simulink model "HIL_Testing_SW"  (Simulink 7.5)
settings: Solver=ode1  StartTime=0.0  StopTime=Inf  FixedStep=0.001  RelTol=1e-3
PostLoadFcn:
  | , if any(exist('dsrtsu_mdlpostloadfcn', 'file') == [2, 3, 6]), try dsrtsu_mdlpostloadfcn('Execute', bdroot); catch fprintf('Error in PostLoadFcn (dsrtsu_mdlpostloadfcn) for model "%s":\n %s\n', bdroot, lasterr); end, end,
undefined symbols (not defined in the file): CeBSER_Cnt_NumTempAxisPts, ChargeCord, ChargeCord_Control, ChargeToSOCCurr, ChrgCurrLim, CrntSens1Fine, CS_SOCSetPt, CyclerMaxChrgPwr, CyclerMaxDschrgPwr, deltaAhr, Drive_1, Drive_10, Drive_11, Drive_12, Drive_13, Drive_14, Drive_15, Drive_16, Drive_17, Drive_18, Drive_19, Drive_2, Drive_20, Drive_21, Drive_22, Drive_23, Drive_24, Drive_25, Drive_26, Drive_27, Drive_28, Drive_29, Drive_3, Drive_30, Drive_31, Drive_32, Drive_33, Drive_34, Drive_35, Drive_36, Drive_37, Drive_38, Drive_39, Drive_4, Drive_40, Drive_41, Drive_42, Drive_43, Drive_44, Drive_45, Drive_46, Drive_47, Drive_48, Drive_49, Drive_5, Drive_50, Drive_51, Drive_6, Drive_7, Drive_8 ... (+50)
libraries: simulink x129, rtican x50, rti2211sailib x5, rti2211serlib x5, rti2202miolib x3
(part 18 of 23)

== system HIL_Testing_SW/LionsHeart/FeaturePresentation/Down_to_Business/DriveProfile_ModeControl/Pulse ==
  Current : Inport  OutDataType=fixdt(1, 16)  OutScaling=2^0
  Voltage : Inport  Port=2  OutDataType=fixdt(1, 16)  OutScaling=2^0
  Direction : Inport  Port=3  OutDataType=fixdt(1, 16)  OutScaling=2^0
  Enable : EnablePort  StatesWhenEnabling=reset
  Data Store Read1 : DataStoreRead  DataStoreName=CyclerMaxDschrgPwr  SampleTime=0
  Data Store Read10 : DataStoreRead  DataStoreName=DschrgCurrLim  SampleTime=0
  Data Store Read2 : DataStoreRead  DataStoreName=CyclerMaxChrgPwr  SampleTime=0
  Data Store Read9 : DataStoreRead  DataStoreName=ChrgCurrLim  SampleTime=0
  Data Type Conversion : DataTypeConversion  OutDataTypeMode=single  OutDataType=sfix(16)  OutScaling=2^0  OutDataTypeStr=single
  Data Type Conversion1 : DataTypeConversion  OutDataTypeMode=single  OutDataType=sfix(16)  OutScaling=2^0  OutDataTypeStr=single
  Pulse : Stateflow chart  TreatAsAtomicUnit=on
  PulseDuration : Constant  Tag=R12-1  Value=10  OutDataTypeMode=double  OutDataType=sfix(16)  OutScaling=2^0  OutDataTypeStr=double
  Terminator2 : Terminator
  simstep : Constant  Tag=R12-1  Value=SimStep_dT  OutDataTypeMode=double  OutDataType=sfix(16)  OutScaling=2^0  OutDataTypeStr=double
  Profile_Data_Pulse : Outport  OutDataType=sfix(16)  OutScaling=2^0
  Mode_Cntrl : Outport  Port=2  OutDataType=sfix(16)  OutScaling=2^0
  PulseStep : Outport  Port=3  OutDataType=sfix(16)  OutScaling=2^0
  wires:
  Current/1 -> [Current]
  Voltage/1 -> [Voltage]
  [Voltage] -> Pulse/1(Voltage)
  [Current] -> Pulse/2(Current)
  simstep/1 -> Data Type Conversion1/1
  Data Type Conversion/1 -> Profile_Data_Pulse/1
  Pulse/3(Mode_Cntrl) -> Mode_Cntrl/1
  Pulse/1(Control_Value) -> Data Type Conversion/1
  Data Type Conversion1/1 -> Pulse/3(sim_step_time)
  Pulse/2(WaitTime) -> Terminator2/1  "Waitime"
  Data Store Read9/1 -> Pulse/4(ChrgCurrLim)
  Data Store Read10/1 -> Pulse/5(DischrgCurrLim)
  Pulse/4(Step) -> PulseStep/1
  Direction/1 -> [direction]
  [direction] -> Pulse/6(Direction)
  Data Store Read1/1 -> Pulse/8(DPower)
  Data Store Read2/1 -> Pulse/7(CPower)
  PulseDuration/1 -> Pulse/9(PulseDuration)

== system HIL_Testing_SW/LionsHeart/FeaturePresentation/Down_to_Business/DriveProfile_ModeControl/Rate ==
  CurrLimit : Inport  OutDataType=fixdt(1, 16)  OutScaling=2^0
  Rate : Inport  Port=2  OutDataType=fixdt(1, 16)  OutScaling=2^0
  Direction : Inport  Port=3  OutDataType=fixdt(1, 16)  OutScaling=2^0
  Enable : EnablePort  StatesWhenEnabling=reset
  Data Store Read10 : DataStoreRead  DataStoreName=DisChrgCurr_Limit  SampleTime=0
  Data Store Read9 : DataStoreRead  DataStoreName=ChargeLimit_Temp  SampleTime=0
  Data Store Write15 : DataStoreWrite  DataStoreName=ChrgCurrLim  SampleTime=-1
  Data Store Write16 : DataStoreWrite  DataStoreName=DschrgCurrLim  SampleTime=-1
  Data Type Conversion1 : DataTypeConversion  OutDataTypeMode=single  OutDataType=sfix(16)  OutScaling=2^0  OutDataTypeStr=single
  PTime : Constant  Value=4  OutDataTypeMode=single  OutDataType=fixdt(1, 16)  OutScaling=2^0  OutDataTypeStr=single
  Product : Product  OutDataType=fixdt(1, 16)  OutScaling=2^0  RndMeth=Zero
  PulseRate : Stateflow chart  TreatAsAtomicUnit=on
  Rate Limiter Dynamic1 : simulink/Discontinuities/Rate Limiter Dynamic  SystemSampleTime=-1
  Rate Limiter Dynamic2 : simulink/Discontinuities/Rate Limiter Dynamic  SystemSampleTime=-1
  Saturation Dynamic : simulink/Discontinuities/Saturation Dynamic  SystemSampleTime=-1  OutMin=[]  OutMax=[]  OutDataTypeStr=single  OutputDataTypeScalingMode=single  OutDataType=sfix(16)  OutScaling=2^-10  DoSatur=off
  Saturation Dynamic1 : simulink/Discontinuities/Saturation Dynamic  SystemSampleTime=-1  OutMin=[]  OutMax=[]  OutDataTypeStr=single  OutputDataTypeScalingMode=single  OutDataType=sfix(16)  OutScaling=2^-10  DoSatur=off
  lolim : Constant  Value=0  OutDataTypeMode=single  OutDataType=fixdt(1, 16)  OutScaling=2^0  OutDataTypeStr=single
  lolim1 : Constant  Value=0  OutDataTypeMode=single  OutDataType=fixdt(1, 16)  OutScaling=2^0  OutDataTypeStr=single
  lolim2 : Constant  Value=-1  OutDataTypeMode=single  OutDataType=fixdt(1, 16)  OutScaling=2^0  OutDataTypeStr=single
  simstep : Constant  Tag=R12-1  Value=SimStep_dT  OutDataTypeMode=double  OutDataType=sfix(16)  OutScaling=2^0  OutDataTypeStr=double
  Profile_Data_rate : Outport  OutDataType=sfix(16)  OutScaling=2^0
  Mode_Cntrl_rate : Outport  Port=2  OutDataType=sfix(16)  OutScaling=2^0
  RateStep : Outport  Port=3  OutDataType=sfix(16)  OutScaling=2^0
  wires:
  Data Type Conversion1/1 -> PulseRate/1(sim_step_time)
  simstep/1 -> Data Type Conversion1/1
  Rate Limiter Dynamic1/1 -> Saturation Dynamic/2
  CurrLimit/1 -> [CurrLimit]
  Rate/1 -> [Rate]
  PulseRate/1(Control_Value) -> Profile_Data_rate/1
  PulseRate/3(Mode_Cntrl) -> Mode_Cntrl_rate/1
  PulseRate/4(Step) -> RateStep/1
  Data Store Read9/1 -> PulseRate/2(ChrgCurrLim_Cal)
  Data Store Read10/1 -> PulseRate/3(DischrgCurrLim_Cal)
  Saturation Dynamic/1 -> Data Store Write15/1
  PulseRate/2(ChrgCurrLim_Temp) -> Saturation Dynamic/1, Rate Limiter Dynamic1/2
  lolim/1 -> Rate Limiter Dynamic1/3, Saturation Dynamic/3
  [Rate] -> Rate Limiter Dynamic1/1
  Direction/1 -> PulseRate/4(Direction)
  PTime/1 -> PulseRate/5(PTime)
  [CurrLimit] -> PulseRate/6(CurrLim)
  Rate Limiter Dynamic2/1 -> Saturation Dynamic1/2
  PulseRate/5(DischrgCurrLim_Temp) -> Rate Limiter Dynamic2/2, Saturation Dynamic1/1
  lolim1/1 -> Rate Limiter Dynamic2/3, Saturation Dynamic1/3
  lolim2/1 -> Product/1
  Saturation Dynamic1/1 -> Product/2
  Product/1 -> Data Store Write16/1
  [Rate] -> Rate Limiter Dynamic2/1

== system HIL_Testing_SW/LionsHeart/FeaturePresentation/Down_to_Business/DriveProfile_ModeControl/Standby_Sub ==
  Enable : EnablePort
  Standby : Constant  Value=single(3)  OutDataType=sfix(16)  OutScaling=2^0
  Standby1 : Outport  OutDataType=fixdt(1, 16)  OutScaling=2^0
  wires:
  Standby/1 -> Standby1/1

== system HIL_Testing_SW/LionsHeart/Input Processing/Voltage Processing/ChargeTermVoltage/ConvCellToPack_Volt1 ==
  note: ConvCellToPack_Volt
  CellLevel_Volt : Inport  OutDataType=sfix(16)  OutScaling=2^0
  Product : Product  OutDataType=sfix(16)  OutScaling=2^0  RndMeth=Zero
  SOCTerm : DataStoreRead  DataStoreName=NumberOfCells  SampleTime=0
  PackLevel_Volt : Outport  OutDataType=sfix(16)  OutScaling=2^0
  wires:
  SOCTerm/1 -> Product/2
  Product/1 -> PackLevel_Volt/1
  CellLevel_Volt/1 -> Product/1

== system HIL_Testing_SW/LionsHeart/Input Processing/Voltage Processing/ChargeTermVoltage/ConvCellToPack_Volt2 ==
  note: ConvCellToPack_Volt
  CellLevel_Volt : Inport  OutDataType=sfix(16)  OutScaling=2^0
  Product : Product  OutDataType=sfix(16)  OutScaling=2^0  RndMeth=Zero
  SOCTerm : DataStoreRead  DataStoreName=NumberOfCells  SampleTime=0
  PackLevel_Volt : Outport  OutDataType=sfix(16)  OutScaling=2^0
  wires:
  CellLevel_Volt/1 -> Product/1
  Product/1 -> PackLevel_Volt/1
  SOCTerm/1 -> Product/2

== system HIL_Testing_SW/LionsHeart/Input Processing/Voltage Processing/ChargeTermVoltage/LookupChrgVoltageSetPoint_BSE ==
  note: LookupChrgVoltageSetPoint
  SocACChrg : Inport  OutDataType=sfix(16)  OutScaling=2^0
  T : Inport  Port=2  OutDataType=sfix(16)  OutScaling=2^0
  Constant Value : Constant  Value=CeBSER_Cnt_NumTempAxisPts  OutDataType=sfix(16)  OutScaling=2^0
  Constant Value1 : Constant  Value=single(100)  OutDataType=sfix(16)  OutScaling=2^0
  KnBSEM_T_TempAxis : Constant  Value=KnBSEM_T_TempAxis  OutDataType=sfix(16)  OutScaling=2^0
      settings: CopyFcn=try,set_param(gcb,'Value',get_param(gcb,'Name'));catch,err=lasterror;if (isempty(strfind(err.message,'Attempting to override parameters')) || isempty(strfind(err.message,'which is inside a library link'))) rethrow(err);end;end  NameChangeFcn=try,set_param(gcb,'Value',get_param(gcb,'Name'));catch,[msgstr msgid]=lasterr;errordlg(['error ',num2str(msgid),' - ',msgstr],'Error','modal');end  OpenFcn=global edarrcal; edarrcal.cb = gcb; edfigarrcal('fig');
  Merge : Merge  Inputs=8
  Product1 : Product  Inputs=*/  OutDataType=sfix(16)  OutScaling=2^0  RndMeth=Zero
  Stateflow Chart1 : Stateflow chart  TreatAsAtomicUnit=on
      settings: CopyFcn=breaklink(gcb)
  Switch Case : SwitchCase  CaseConditions={1,2,3,4,5,6,7,8}  ShowDefaultCase=off
      settings: CopyFcn=breaklink(gcb)
  Switch Case Action Subsystem : Subsystem  TreatAsAtomicUnit=on
      settings: CopyFcn=breaklink(gcb)  PropExecContextOutsideSubsystem=on
  Switch Case Action Subsystem1 : Subsystem  TreatAsAtomicUnit=on
      settings: CopyFcn=breaklink(gcb)  PropExecContextOutsideSubsystem=on
  Switch Case Action Subsystem2 : Subsystem  TreatAsAtomicUnit=on
      settings: CopyFcn=breaklink(gcb)  PropExecContextOutsideSubsystem=on
  Switch Case Action Subsystem3 : Subsystem  TreatAsAtomicUnit=on
      settings: CopyFcn=breaklink(gcb)  PropExecContextOutsideSubsystem=on
  Switch Case Action Subsystem4 : Subsystem  TreatAsAtomicUnit=on
      settings: CopyFcn=breaklink(gcb)  PropExecContextOutsideSubsystem=on
  Switch Case Action Subsystem5 : Subsystem  TreatAsAtomicUnit=on
      settings: CopyFcn=breaklink(gcb)  PropExecContextOutsideSubsystem=on
  Switch Case Action Subsystem6 : Subsystem  TreatAsAtomicUnit=on
      settings: CopyFcn=breaklink(gcb)  PropExecContextOutsideSubsystem=on
  Switch Case Action Subsystem7 : Subsystem  TreatAsAtomicUnit=on
      settings: CopyFcn=breaklink(gcb)  PropExecContextOutsideSubsystem=on
  Output Parameter : Outport  OutDataType=sfix(16)  OutScaling=2^0
  wires:
  SocACChrg/1 -> Product1/1
  Product1/1 -> [SOC]
  Constant Value1/1 -> Product1/2
  Switch Case Action Subsystem7/1(Output Parameter) -> Merge/8
  Switch Case Action Subsystem6/1(Output Parameter) -> Merge/7
  Switch Case Action Subsystem5/1(Output Parameter) -> Merge/6
  Switch Case Action Subsystem4/1(Output Parameter) -> Merge/5
  Switch Case Action Subsystem3/1(Output Parameter) -> Merge/4
  Switch Case Action Subsystem2/1(Output Parameter) -> Merge/3
  Switch Case Action Subsystem1/1(Output Parameter) -> Merge/2
  Switch Case Action Subsystem/1(Output Parameter) -> Merge/1
  T/1 -> Stateflow Chart1/1(VeBSER_T_HV_BatTemp)
  [Idx8] -> Switch Case Action Subsystem7/Action
  [SOC] -> Switch Case Action Subsystem7/1(SOC)
  [SF] -> Switch Case Action Subsystem7/2(SF)
  [Idx7] -> Switch Case Action Subsystem6/Action
  [SOC] -> Switch Case Action Subsystem6/1(SOC)
  [SF] -> Switch Case Action Subsystem6/2(SF)
  [Idx6] -> Switch Case Action Subsystem5/Action
  [SOC] -> Switch Case Action Subsystem5/1(SOC)
  [SF] -> Switch Case Action Subsystem5/2(SF)
  [Idx5] -> Switch Case Action Subsystem4/Action
  [SOC] -> Switch Case Action Subsystem4/1(SOC)
  [SF] -> Switch Case Action Subsystem4/2(SF)
  [Idx4] -> Switch Case Action Subsystem3/Action
  [SOC] -> Switch Case Action Subsystem3/1(SOC)
  [SF] -> Switch Case Action Subsystem3/2(SF)
  [Idx3] -> Switch Case Action Subsystem2/Action
  [SOC] -> Switch Case Action Subsystem2/1(SOC)
  [SF] -> Switch Case Action Subsystem2/2(SF)
  [Idx2] -> Switch Case Action Subsystem1/Action
  [SOC] -> Switch Case Action Subsystem1/1(SOC)
  [SF] -> Switch Case Action Subsystem1/2(SF)
  Merge/1 -> Output Parameter/1
  [Idx1] -> Switch Case Action Subsystem/Action
  Switch Case/8 -> [Idx8]
  Switch Case/7 -> [Idx7]
  Switch Case/6 -> [Idx6]
  Switch Case/5 -> [Idx5]
  Switch Case/4 -> [Idx4]
  Switch Case/3 -> [Idx3]
  Switch Case/2 -> [Idx2]
  Switch Case/1 -> [Idx1]
  Stateflow Chart1/1(LeBSER_i_Indx) -> Switch Case/1
  KnBSEM_T_TempAxis/1 -> Stateflow Chart1/2(KnBSEM_T_TempAxis)
  Stateflow Chart1/2(LeBSER_r_ScaleFctr) -> [SF]
  [SOC] -> Switch Case Action Subsystem/1(SOC)
  [SF] -> Switch Case Action Subsystem/2(SF)
  Constant Value/1 -> Stateflow Chart1/3(CeBSER_Cnt_NumTempAxisPts)

== system HIL_Testing_SW/LionsHeart/Input Processing/Voltage Processing/PackVLid/ConvCellToPack_Volt4 ==
  note: ConvCellToPack_Volt
  CellLevel_Volt : Inport  OutDataType=sfix(16)  OutScaling=2^0
  NumberOfCells : DataStoreRead  DataStoreName=NumberOfCells  SampleTime=0
  Product : Product  OutDataType=sfix(16)  OutScaling=2^0  RndMeth=Zero
  PackLevel_Volt : Outport  OutDataType=sfix(16)  OutScaling=2^0
  wires:
  CellLevel_Volt/1 -> Product/1
  Product/1 -> PackLevel_Volt/1
  NumberOfCells/1 -> Product/2

== system HIL_Testing_SW/LionsHeart/Input Processing/Voltage Processing/PackVfloor/ConvCellToPack_Volt3 ==
  note: ConvCellToPack_Volt
  CellLevel_Volt : Inport  OutDataType=sfix(16)  OutScaling=2^0
  NumberOfCells : DataStoreRead  DataStoreName=NumberOfCells  SampleTime=0
  Product : Product  OutDataType=sfix(16)  OutScaling=2^0  RndMeth=Zero
  PackLevel_Volt : Outport  OutDataType=sfix(16)  OutScaling=2^0
  wires:
  NumberOfCells/1 -> Product/2
  Product/1 -> PackLevel_Volt/1
  CellLevel_Volt/1 -> Product/1

== system HIL_Testing_SW/LionsHeart/Input Processing/Voltage Processing/PackVfloor/EREV ==
  MinCellOffset : Inport  OutDataType=fixdt(1, 16)  OutScaling=2^0
  MinSectionOffset : Inport  Port=2  OutDataType=fixdt(1, 16)  OutScaling=2^0
  Enable : EnablePort
  Data Store Read : DataStoreRead  DataStoreName=MinSectionorMinCellOffset_EREV  SampleTime=0
  Switch1 : Switch  Threshold=.5  OutDataType=fixdt(1, 16)  OutScaling=2^0
  VoltageFloorOffset_EREV : Outport  OutDataType=fixdt(1, 16)  OutScaling=2^0
  wires:
  MinCellOffset/1 -> Switch1/1
  MinSectionOffset/1 -> Switch1/3
  Switch1/1 -> VoltageFloorOffset_EREV/1
  Data Store Read/1 -> Switch1/2

== system HIL_Testing_SW/LionsHeart/Input Processing/Voltage Processing/PackVfloor/Subsystem1 ==
  MinCellOffset : Inport  OutDataType=fixdt(1, 16)  OutScaling=2^0
  Enable : EnablePort
  VoltageFloorOffset : Outport  OutDataType=fixdt(1, 16)  OutScaling=2^0
  wires:
  MinCellOffset/1 -> VoltageFloorOffset/1

== system HIL_Testing_SW/RTI Data/RTI Data Store/RTI Data Store/RTI Data Store/RTI Data Store ==

== system HIL_Testing_SW/RX/Read EREV/Read HVEM/Current/Enabled Subsystem ==
  SensTwo : Inport  OutDataType=sfix(16)  OutScaling=2^0
  SensOne : Inport  Port=2  OutDataType=sfix(16)  OutScaling=2^0
  Enable : EnablePort
  Abs : Abs  OutDataType=fixdt(1, 16)  OutScaling=2^0
  Switch : Switch  Threshold=20  OutDataType=sfix(16)  OutScaling=2^0
  Out1 : Outport  OutDataType=sfix(16)  OutScaling=2^0
  wires:
  SensTwo/1 -> Switch/1
  Switch/1 -> Out1/1
  SensOne/1 -> Switch/3, Abs/1
  Abs/1 -> Switch/2

== system HIL_Testing_SW/RX/Read EREV/Read HVEM/Current/Enabled Subsystem1 ==
  SensTwo : Inport  OutDataType=sfix(16)  OutScaling=2^0
  SensOne : Inport  Port=2  OutDataType=sfix(16)  OutScaling=2^0
  Enable : EnablePort
  Abs : Abs  OutDataType=fixdt(1, 16)  OutScaling=2^0
  Switch : Switch  Threshold=20  OutDataType=sfix(16)  OutScaling=2^0
  Out1 : Outport  OutDataType=sfix(16)  OutScaling=2^0
  wires:
  Switch/1 -> Out1/1
  SensOne/1 -> Switch/1
  SensTwo/1 -> Switch/3, Abs/1
  Abs/1 -> Switch/2

== system HIL_Testing_SW/RX/Read EREV/Read HVEM/Sum of Cells/Subsystem ==
  In1 : Inport  OutDataType=fixdt(1, 16)  OutScaling=2^0
  Bus Creator : BusCreator  Inputs=42
  Bus Creator1 : BusCreator  Inputs=24
  Bus Creator2 : BusCreator  Inputs=30
  Bus Selector : BusSelector  OutputSignals=signal1.HVBatCell_003,signal1.HVBatCell_006,signal1.HVBatCell_009,signal1.HVBatCell_012,signal1.HVBatCell_015,signal1.HVBatCell_018,signal1.HVBatCell_021,signal1.HVBatCell_024,signal1.HVBatCell_002,signal1.HVBatCell_005,signal1.HVBatCell_008,signal1.HVBatCell_011,signal1.HVBatCell_014,signal1.HVBatCell_017,signal1.HVBatCell_020,signal1.HVBatCell_023,signal1.HVBatCell_001,signal1.HVBatCell_004,signal1.HVBatCell_007,signal1.HVBatCell_010,signal1.HVBatCell_013,signal1.HVBatCell_016,signal1.HVBatCell_019,signal1.HVBatCell_022,signal2.HVBatCell_027,signal2.HVBatCell_030,signal2.HVBatCell_033,signal2.HVBatCell_036,signal2.HVBatCell_039,signal2.HVBatCell_042,signal2.HVBatCell_026,signal2.HVBatCell_029,signal2.HVBatCell_032,signal2.HVBatCell_035,signal2.HVBatCell_038,signal2.HVBatCell_041,signal2.HVBatCell_025,signal2.HVBatCell_028,signal2.HVBatCell_031,signal2.HVBatCell_034,signal2.HVBatCell_037,signal2.HVBatCell_040
  Bus Selector1 : BusSelector  OutputSignals=signal2.HVBatCell_045,signal2.HVBatCell_048,signal2.HVBatCell_044,signal2.HVBatCell_047,signal2.HVBatCell_043,signal2.HVBatCell_046,signal3.HVBatCell_051,signal3.HVBatCell_054,signal3.HVBatCell_057,signal3.HVBatCell_060,signal3.HVBatCell_063,signal3.HVBatCell_066,signal3.HVBatCell_050,signal3.HVBatCell_053,signal3.HVBatCell_056,signal3.HVBatCell_059,signal3.HVBatCell_062,signal3.HVBatCell_065,signal3.HVBatCell_049,signal3.HVBatCell_052,signal3.HVBatCell_055,signal3.HVBatCell_058,signal3.HVBatCell_061,signal3.HVBatCell_064
  Bus Selector2 : BusSelector  OutputSignals=signal3.HVBatCell_069,signal3.HVBatCell_072,signal3.HVBatCell_068,signal3.HVBatCell_071,signal3.HVBatCell_067,signal3.HVBatCell_070,signal4.HVBatCell_075,signal4.HVBatCell_078,signal4.HVBatCell_081,signal4.HVBatCell_084,signal4.HVBatCell_087,signal4.HVBatCell_090,signal4.HVBatCell_093,signal4.HVBatCell_096,signal4.HVBatCell_074,signal4.HVBatCell_077,signal4.HVBatCell_080,signal4.HVBatCell_083,signal4.HVBatCell_086,signal4.HVBatCell_089,signal4.HVBatCell_092,signal4.HVBatCell_095,signal4.HVBatCell_073,signal4.HVBatCell_076,signal4.HVBatCell_079,signal4.HVBatCell_082,signal4.HVBatCell_085,signal4.HVBatCell_088,signal4.HVBatCell_091,signal4.HVBatCell_094
  Divide : Product  Inputs=*/  OutDataType=fixdt(1, 16)  OutScaling=2^-10
  Divide1 : Product  Inputs=*/  OutDataType=fixdt(1, 16)  OutScaling=2^-10
  Divide2 : Product  Inputs=*/  OutDataType=fixdt(1, 16)  OutScaling=2^-10
  MinMax : MinMax  Inputs=3  OutDataType=fixdt(1, 16)  OutScaling=2^0
  NumCells : Constant  Value=42  OutDataType=fixdt(1, 16)  OutScaling=2^0
  NumCells1 : Constant  Value=24  OutDataType=fixdt(1, 16)  OutScaling=2^0
  NumCells2 : Constant  Value=30  OutDataType=fixdt(1, 16)  OutScaling=2^0
  NumOfCells : DataStoreRead  DataStoreName=NumberOfCells  SampleTime=0
  Product : Product  OutDataType=fixdt(1, 16)  OutScaling=2^0  RndMeth=Zero
  Product1 : Product  OutDataType=fixdt(1, 16)  OutScaling=2^0  RndMeth=Zero
  Product2 : Product  OutDataType=fixdt(1, 16)  OutScaling=2^0  RndMeth=Zero
  Sum : Sum  Inputs=+  OutDataType=fixdt(1, 16)  OutScaling=2^-10
  Sum1 : Sum  Inputs=+  OutDataType=fixdt(1, 16)  OutScaling=2^-10
  Sum2 : Sum  Inputs=+  OutDataType=fixdt(1, 16)  OutScaling=2^-10
  MinSection_PackEquivalent : Outport  OutDataType=fixdt(1, 16)  OutScaling=2^0
  wires:
  In1/1 -> Bus Selector/1, Bus Selector1/1, Bus Selector2/1
  Bus Creator/1 -> Sum/1
  Sum/1 -> Divide/1
  NumCells/1 -> Divide/2
  Divide/1 -> Product/1
  Bus Selector/1 -> Bus Creator/1  "<HVBatCell_003>"
  Bus Selector/2 -> Bus Creator/2  "<HVBatCell_006>"
  Bus Selector/3 -> Bus Creator/3  "<HVBatCell_009>"
  Bus Selector/4 -> Bus Creator/4  "<HVBatCell_012>"
  Bus Selector/5 -> Bus Creator/5  "<HVBatCell_015>"
  Bus Selector/6 -> Bus Creator/6  "<HVBatCell_018>"
  Bus Selector/7 -> Bus Creator/7  "<HVBatCell_021>"
  Bus Selector/8 -> Bus Creator/8  "<HVBatCell_024>"
  Bus Selector/9 -> Bus Creator/9  "<HVBatCell_002>"
  Bus Selector/10 -> Bus Creator/10  "<HVBatCell_005>"
  Bus Selector/11 -> Bus Creator/11  "<HVBatCell_008>"
  Bus Selector/12 -> Bus Creator/12  "<HVBatCell_011>"
  Bus Selector/13 -> Bus Creator/13  "<HVBatCell_014>"
  Bus Selector/14 -> Bus Creator/14  "<HVBatCell_017>"
  Bus Selector/15 -> Bus Creator/15  "<HVBatCell_020>"
  Bus Selector/16 -> Bus Creator/16  "<HVBatCell_023>"
  Bus Selector/17 -> Bus Creator/17  "<HVBatCell_001>"
  Bus Selector/18 -> Bus Creator/18  "<HVBatCell_004>"
  Bus Selector/19 -> Bus Creator/19  "<HVBatCell_007>"
  Bus Selector/20 -> Bus Creator/20  "<HVBatCell_010>"
  Bus Selector/21 -> Bus Creator/21  "<HVBatCell_013>"
  Bus Selector/22 -> Bus Creator/22  "<HVBatCell_016>"
  Bus Selector/23 -> Bus Creator/23  "<HVBatCell_019>"
  Bus Selector/24 -> Bus Creator/24  "<HVBatCell_022>"
  Bus Selector/25 -> Bus Creator/25  "<HVBatCell_027>"
  Bus Selector/26 -> Bus Creator/26  "<HVBatCell_030>"
  Bus Selector/27 -> Bus Creator/27  "<HVBatCell_033>"
  Bus Selector/28 -> Bus Creator/28  "<HVBatCell_036>"
  Bus Selector/29 -> Bus Creator/29  "<HVBatCell_039>"
  Bus Selector/30 -> Bus Creator/30  "<HVBatCell_042>"
  Bus Selector/31 -> Bus Creator/31  "<HVBatCell_026>"
  Bus Selector/32 -> Bus Creator/32  "<HVBatCell_029>"
  Bus Selector/33 -> Bus Creator/33  "<HVBatCell_032>"
  Bus Selector/34 -> Bus Creator/34  "<HVBatCell_035>"
  Bus Selector/35 -> Bus Creator/35  "<HVBatCell_038>"
  Bus Selector/36 -> Bus Creator/36  "<HVBatCell_041>"
  Bus Selector/37 -> Bus Creator/37  "<HVBatCell_025>"
  Bus Selector/38 -> Bus Creator/38  "<HVBatCell_028>"
  Bus Selector/39 -> Bus Creator/39  "<HVBatCell_031>"
  Bus Selector/40 -> Bus Creator/40  "<HVBatCell_034>"
  Bus Selector/41 -> Bus Creator/41  "<HVBatCell_037>"
  Bus Selector/42 -> Bus Creator/42  "<HVBatCell_040>"
  NumOfCells/1 -> [NumberOfCells]
  [NumberOfCells] -> Product/2
  Bus Selector1/1 -> Bus Creator1/1  "<HVBatCell_045>"
  Bus Selector1/2 -> Bus Creator1/2  "<HVBatCell_048>"
  Bus Selector1/3 -> Bus Creator1/3  "<HVBatCell_044>"
  Bus Selector1/4 -> Bus Creator1/4  "<HVBatCell_047>"
  Bus Selector1/5 -> Bus Creator1/5  "<HVBatCell_043>"
  Bus Selector1/6 -> Bus Creator1/6  "<HVBatCell_046>"
  Bus Selector1/7 -> Bus Creator1/7  "<HVBatCell_051>"
  Bus Selector1/8 -> Bus Creator1/8  "<HVBatCell_054>"
  Bus Selector1/9 -> Bus Creator1/9  "<HVBatCell_057>"
  Bus Selector1/10 -> Bus Creator1/10  "<HVBatCell_060>"
  Bus Selector1/11 -> Bus Creator1/11  "<HVBatCell_063>"
  Bus Selector1/12 -> Bus Creator1/12  "<HVBatCell_066>"
  Bus Selector1/13 -> Bus Creator1/13  "<HVBatCell_050>"
  Bus Selector1/14 -> Bus Creator1/14  "<HVBatCell_053>"
  Bus Selector1/15 -> Bus Creator1/15  "<HVBatCell_056>"
  Bus Selector1/16 -> Bus Creator1/16  "<HVBatCell_059>"
  Bus Selector1/17 -> Bus Creator1/17  "<HVBatCell_062>"
  Bus Selector1/18 -> Bus Creator1/18  "<HVBatCell_065>"
  Bus Selector1/19 -> Bus Creator1/19  "<HVBatCell_049>"
  Bus Selector1/20 -> Bus Creator1/20  "<HVBatCell_052>"
  Bus Selector1/21 -> Bus Creator1/21  "<HVBatCell_055>"
  Bus Selector1/22 -> Bus Creator1/22  "<HVBatCell_058>"
  Bus Selector1/23 -> Bus Creator1/23  "<HVBatCell_061>"
  Bus Selector1/24 -> Bus Creator1/24  "<HVBatCell_064>"
  Bus Creator1/1 -> Sum1/1
  Sum1/1 -> Divide1/1
  NumCells1/1 -> Divide1/2
  Divide1/1 -> Product1/1
  [NumberOfCells] -> Product1/2
  Bus Selector2/1 -> Bus Creator2/1  "<HVBatCell_069>"
  Bus Selector2/2 -> Bus Creator2/2  "<HVBatCell_072>"
  Bus Selector2/3 -> Bus Creator2/3  "<HVBatCell_068>"
  Bus Selector2/4 -> Bus Creator2/4  "<HVBatCell_071>"
  Bus Selector2/5 -> Bus Creator2/5  "<HVBatCell_067>"
  Bus Selector2/6 -> Bus Creator2/6  "<HVBatCell_070>"
  Bus Selector2/7 -> Bus Creator2/7  "<HVBatCell_075>"
  Bus Selector2/8 -> Bus Creator2/8  "<HVBatCell_078>"
  Bus Selector2/9 -> Bus Creator2/9  "<HVBatCell_081>"
  Bus Selector2/10 -> Bus Creator2/10  "<HVBatCell_084>"
  Bus Selector2/11 -> Bus Creator2/11  "<HVBatCell_087>"
  Bus Selector2/12 -> Bus Creator2/12  "<HVBatCell_090>"
  Bus Selector2/13 -> Bus Creator2/13  "<HVBatCell_093>"
  Bus Selector2/14 -> Bus Creator2/14  "<HVBatCell_096>"
  Bus Selector2/15 -> Bus Creator2/15  "<HVBatCell_074>"
  Bus Selector2/16 -> Bus Creator2/16  "<HVBatCell_077>"
  Bus Selector2/17 -> Bus Creator2/17  "<HVBatCell_080>"
  Bus Selector2/18 -> Bus Creator2/18  "<HVBatCell_083>"
  Bus Selector2/19 -> Bus Creator2/19  "<HVBatCell_086>"
  Bus Selector2/20 -> Bus Creator2/20  "<HVBatCell_089>"
  Bus Selector2/21 -> Bus Creator2/21  "<HVBatCell_092>"
  Bus Selector2/22 -> Bus Creator2/22  "<HVBatCell_095>"
  Bus Selector2/23 -> Bus Creator2/23  "<HVBatCell_073>"
  Bus Selector2/24 -> Bus Creator2/24  "<HVBatCell_076>"
  Bus Selector2/25 -> Bus Creator2/25  "<HVBatCell_079>"
  Bus Selector2/26 -> Bus Creator2/26  "<HVBatCell_082>"
  Bus Selector2/27 -> Bus Creator2/27  "<HVBatCell_085>"
  Bus Selector2/28 -> Bus Creator2/28  "<HVBatCell_088>"
  Bus Selector2/29 -> Bus Creator2/29  "<HVBatCell_091>"
  Bus Selector2/30 -> Bus Creator2/30  "<HVBatCell_094>"
  Bus Creator2/1 -> Sum2/1
  Sum2/1 -> Divide2/1
  NumCells2/1 -> Divide2/2
  Divide2/1 -> Product2/1
  [NumberOfCells] -> Product2/2
  Product/1 -> MinMax/1
  Product1/1 -> MinMax/2
  Product2/1 -> MinMax/3
  MinMax/1 -> MinSection_PackEquivalent/1

== system HIL_Testing_SW/TX/Chiller/ChillerCmndTxDecision/ChillerRxProcessing/ChillerPositiveResponse ==
  Action Port : ActionPort  ActionType=elseif
  Compare To Constant : simulink/Logic and Bit Operations/Compare To Constant  SystemSampleTime=-1  relop===  const=33  LogicOutDataTypeMode=boolean
  Compare To Constant1 : simulink/Logic and Bit Operations/Compare To Constant  SystemSampleTime=-1  relop===  const=13  LogicOutDataTypeMode=boolean
  Data Store Read1 : DataStoreRead  DataStoreName=RxChillerFIFO  SampleTime=-1
  Demux : Demux  Outputs=7
  Logical Operator : Logic  AllPortsSameDT=off  OutDataTypeMode=boolean  LogicDataType=fixdt(0, 8)  OutDataTypeStr=boolean
  Terminator{1,3..6} (5 alike) : Terminator
  ChillerPositiveResponse : Outport
  wires:
  [RxByteOne] -> Compare To Constant/1
  [RxByteTwo] -> Compare To Constant1/1
  Compare To Constant1/1 -> Logical Operator/2
  Compare To Constant/1 -> Logical Operator/1
  Logical Operator/1 -> ChillerPositiveResponse/1  "ChillerPositiveResponse"
  Demux/1 -> [RxByteOne]
  Demux/3 -> Terminator1/1
  Demux/4 -> Terminator3/1
  Demux/6 -> Terminator5/1
  Data Store Read1/1 -> Demux/1
  Demux/2 -> [RxByteTwo]
  Demux/5 -> Terminator4/1
  Demux/7 -> Terminator6/1

== system HIL_Testing_SW/TX/Chiller/ChillerCmndTxDecision/ChillerRxProcessing/ChillerStatus ==
  Action Port : ActionPort  ActionType=elseif
  Compare To Constant : simulink/Logic and Bit Operations/Compare To Constant  SystemSampleTime=-1  relop===  const=49  LogicOutDataTypeMode=boolean
  Compare To Constant1 : simulink/Logic and Bit Operations/Compare To Constant  SystemSampleTime=-1  relop===  const=13  LogicOutDataTypeMode=boolean
  Data Store Read1 : DataStoreRead  DataStoreName=RxChillerFIFO  SampleTime=-1
  Demux : Demux  Outputs=7
  Logical Operator : Logic  AllPortsSameDT=off  OutDataTypeMode=boolean  LogicDataType=fixdt(0, 8)  OutDataTypeStr=boolean
  Terminator{1,3..6} (5 alike) : Terminator
  ChillerOn : Outport
  wires:
  Demux/7 -> Terminator6/1
  Demux/5 -> Terminator4/1
  Demux/2 -> [RxByteTwo]
  Data Store Read1/1 -> Demux/1
  Demux/6 -> Terminator5/1
  Demux/4 -> Terminator3/1
  Demux/3 -> Terminator1/1
  Demux/1 -> [RxByteOne]
  Logical Operator/1 -> ChillerOn/1  "ChillerOn"
  Compare To Constant/1 -> Logical Operator/1
  Compare To Constant1/1 -> Logical Operator/2
  [RxByteTwo] -> Compare To Constant1/1
  [RxByteOne] -> Compare To Constant/1

== system HIL_Testing_SW/TX/Chiller/ChillerCmndTxDecision/ChillerRxProcessing/ReadChillerSP ==
  NumRxBytes : Inport  OutDataType=fixdt(1, 16)  OutScaling=2^0
  Action Port : ActionPort  ActionType=then
  Compare To Constant : simulink/Logic and Bit Operations/Compare To Constant  SystemSampleTime=-1  relop===  const=7  LogicOutDataTypeMode=boolean
  Compare To Constant1 : simulink/Logic and Bit Operations/Compare To Constant  SystemSampleTime=-1  relop===  const=4  LogicOutDataTypeMode=boolean
  Gain : Gain  ParameterDataType=fixdt(1, 16)  ParameterScaling=2^0  OutDataType=fixdt(1, 16)  OutScaling=2^0
  If : If  NumInputs=2  IfExpression=u1 == 1  ElseIfExpressions=u2 == 1  ShowElse=off
  Merge : Merge
  RxReadChillerSP4Bytes : Subsystem  TreatAsAtomicUnit=on
  RxReadChillerSP7Bytes : Subsystem  TreatAsAtomicUnit=on
  RxReadChillerSetPoint : Outport  OutDataType=fixdt(1, 16)  OutScaling=2^0
  wires:
  NumRxBytes/1 -> Compare To Constant/1, Compare To Constant1/1
  Compare To Constant/1 -> If/1
  Compare To Constant1/1 -> If/2
  If/1 -> RxReadChillerSP7Bytes/Action
  RxReadChillerSP7Bytes/1(RxReadChillerSetPoint) -> Merge/1
  RxReadChillerSP4Bytes/1(RxReadChillerSetPoint) -> Merge/2
  If/2 -> RxReadChillerSP4Bytes/Action
  Merge/1 -> Gain/1
  Gain/1 -> RxReadChillerSetPoint/1  "ReadChillerSP"

== system HIL_Testing_SW/TX/Chiller/ChillerCmndTxDecision/ChillerRxProcessing/ReadChillerTemp ==
  NumRxBytes : Inport  OutDataType=fixdt(1, 16)  OutScaling=2^0
  Action Port : ActionPort  ActionType=elseif
  Compare To Constant : simulink/Logic and Bit Operations/Compare To Constant  SystemSampleTime=-1  relop===  const=7  LogicOutDataTypeMode=boolean
  Compare To Constant1 : simulink/Logic and Bit Operations/Compare To Constant  SystemSampleTime=-1  relop===  const=4  LogicOutDataTypeMode=boolean
  Gain : Gain  ParameterDataType=fixdt(1, 16)  ParameterScaling=2^0  OutDataType=fixdt(1, 16)  OutScaling=2^0
  If : If  NumInputs=2  IfExpression=u1 == 1  ElseIfExpressions=u2 == 1  ShowElse=off
  Merge : Merge
  RxReadChillerTemp4Bytes : Subsystem  TreatAsAtomicUnit=on
  RxReadChillerTemp7Bytes : Subsystem  TreatAsAtomicUnit=on
  RxReadChillerTemp : Outport  OutDataType=fixdt(1, 16)  OutScaling=2^0
  wires:
  NumRxBytes/1 -> Compare To Constant/1, Compare To Constant1/1
  Compare To Constant/1 -> If/1
  Compare To Constant1/1 -> If/2
  If/1 -> RxReadChillerTemp7Bytes/Action
  RxReadChillerTemp7Bytes/1(RxReadChillerSetPoint) -> Merge/1
  RxReadChillerTemp4Bytes/1(RxReadChillerSetPoint) -> Merge/2
  If/2 -> RxReadChillerTemp4Bytes/Action
  Merge/1 -> Gain/1
  Gain/1 -> RxReadChillerTemp/1  "RxReadChillerTemp"

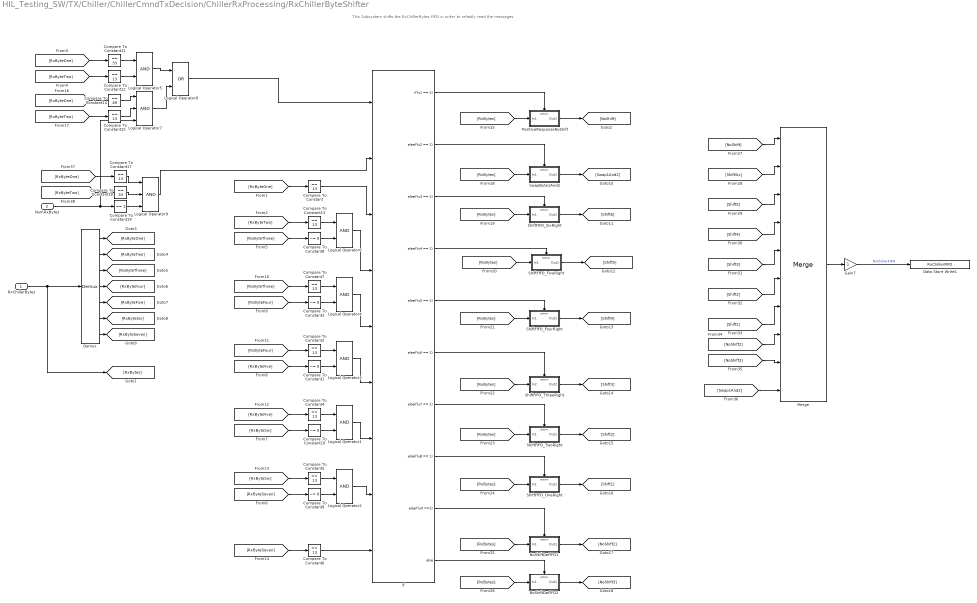
== system HIL_Testing_SW/TX/Chiller/ChillerCmndTxDecision/ChillerRxProcessing/RxChillerByteShifter ==
  note: This Subsystem shifts the RxChillerBytes
      |       FIFO in order to reliably read the messages.
  RxChillerBytes : Inport  OutDataType=fixdt(1, 16)  OutScaling=2^0
  NumRxBytes : Inport  Port=2  OutDataType=fixdt(1, 16)  OutScaling=2^0
  Compare To Constant{,2,4..7,12..13,15,17} (10 alike) : simulink/Logic and Bit Operations/Compare To Constant  SystemSampleTime=-1  relop===  const=13  LogicOutDataTypeMode=boolean
  Compare To Constant{1,3,8..10} (5 alike) : simulink/Logic and Bit Operations/Compare To Constant  SystemSampleTime=-1  relop=~=  const=0  LogicOutDataTypeMode=boolean
  Compare To Constant11 : simulink/Logic and Bit Operations/Compare To Constant  SystemSampleTime=-1  relop===  const=33  LogicOutDataTypeMode=boolean
  Compare To Constant14 : simulink/Logic and Bit Operations/Compare To Constant  SystemSampleTime=-1  relop===  const=49  LogicOutDataTypeMode=boolean
  Compare To Constant18 : simulink/Logic and Bit Operations/Compare To Constant  SystemSampleTime=-1  relop===  const=33  LogicOutDataTypeMode=boolean
  Compare To Constant19 : simulink/Logic and Bit Operations/Compare To Constant  SystemSampleTime=-1  relop===  const=2  LogicOutDataTypeMode=boolean
  Data Store Write1 : DataStoreWrite  DataStoreName=RxChillerFIFO  SampleTime=-1
  Demux : Demux  Outputs=7
  Gain7 : Gain  ParameterDataType=fixdt(1, 16)  ParameterScaling=2^0  OutDataTypeMode=uint8  OutDataType=fixdt(1, 16)  OutScaling=2^0  OutDataTypeStr=uint8
  If : If  NumInputs=9  IfExpression=u1 == 1  ElseIfExpressions=u2 == 1, u3 == 1, u4 == 1, u5 == 1, u6 == 1, u7 == 1, u8 == 1, u9 ==1
  Logical Operator{1..6} (6 alike) : Logic  AllPortsSameDT=off  OutDataTypeMode=boolean  LogicDataType=fixdt(0, 8)  OutDataTypeStr=boolean
  Logical Operator7 : Logic  Inputs=3  AllPortsSameDT=off  OutDataTypeMode=boolean  LogicDataType=fixdt(0, 8)  OutDataTypeStr=boolean
  Logical Operator8 : Logic  Operator=OR  AllPortsSameDT=off  OutDataTypeMode=boolean  LogicDataType=fixdt(0, 8)  OutDataTypeStr=boolean
  Logical Operator9 : Logic  Inputs=3  AllPortsSameDT=off  OutDataTypeMode=boolean  LogicDataType=fixdt(0, 8)  OutDataTypeStr=boolean
  Merge : Merge  Inputs=10
  NoShiftDaFIFO1 : Subsystem  TreatAsAtomicUnit=on
  NoShiftDaFIFO2 : Subsystem  TreatAsAtomicUnit=on
  PositiveResponseNoShift : Subsystem  TreatAsAtomicUnit=on
  ShiftFIFO_FiveRight : Subsystem  TreatAsAtomicUnit=on
  ShiftFIFO_FourRight : Subsystem  TreatAsAtomicUnit=on
  ShiftFIFO_OneRight : Subsystem  TreatAsAtomicUnit=on
  ShiftFIFO_SixRight : Subsystem  TreatAsAtomicUnit=on
  ShiftFIFO_ThreeRight : Subsystem  TreatAsAtomicUnit=on
  ShiftFIFO_TwoRight : Subsystem  TreatAsAtomicUnit=on
  SwapByte1And2 : Subsystem  TreatAsAtomicUnit=on
  wires:
  Demux/1 -> [RxByteOne]
  Demux/2 -> [RxByteTwo]
  Demux/3 -> [RxByteThree]
  Demux/4 -> [RxByteFour]
  Demux/5 -> [RxByteFive]
  Demux/6 -> [RxByteSix]
  Demux/7 -> [RxByteSeven]
  RxChillerBytes/1 -> Demux/1, [RxBytes]
  [RxByteOne] -> Compare To Constant/1
  [RxByteSix] -> Compare To Constant5/1
  [RxByteSeven] -> Compare To Constant6/1
  Merge/1 -> Gain7/1
  Gain7/1 -> Data Store Write1/1  "RxChillerFIFO"
  [RxByteFive] -> Compare To Constant4/1
  Compare To Constant4/1 -> Logical Operator1/1
  Compare To Constant5/1 -> Logical Operator2/1
  Compare To Constant9/1 -> Logical Operator2/2
  Compare To Constant11/1 -> Logical Operator5/1
  [RxByteOne] -> Compare To Constant11/1
  [RxByteTwo] -> Compare To Constant12/1
  Compare To Constant12/1 -> Logical Operator5/2
  [RxByteSeven] -> Compare To Constant9/1
  Compare To Constant10/1 -> Logical Operator1/2
  [RxByteSix] -> Compare To Constant10/1
  Compare To Constant2/1 -> Logical Operator3/1
  Compare To Constant1/1 -> Logical Operator3/2
  [RxByteFive] -> Compare To Constant1/1
  [RxByteFour] -> Compare To Constant2/1
  Compare To Constant7/1 -> Logical Operator4/1
  Compare To Constant3/1 -> Logical Operator4/2
  [RxByteThree] -> Compare To Constant7/1
  [RxByteFour] -> Compare To Constant3/1
  Compare To Constant13/1 -> Logical Operator6/1
  Compare To Constant8/1 -> Logical Operator6/2
  [RxByteTwo] -> Compare To Constant13/1
  [RxByteThree] -> Compare To Constant8/1
  If/1 -> PositiveResponseNoShift/Action
  [RxBytes] -> PositiveResponseNoShift/1(In1)
  [RxBytes] -> ShiftFIFO_SixRight/1(In1)
  [RxBytes] -> ShiftFIFO_FiveRight/1(In1)
  [RxBytes] -> ShiftFIFO_FourRight/1(In1)
  [RxBytes] -> ShiftFIFO_ThreeRight/1(In2)
  [RxBytes] -> ShiftFIFO_TwoRight/1(In1)
  [RxBytes] -> ShiftFIFO_OneRight/1(In1)
  [RxBytes] -> NoShiftDaFIFO1/1(In1)
  PositiveResponseNoShift/1(Out1) -> [NoShift]
  [NoShift] -> Merge/1
  [ShiftSix] -> Merge/2
  [Shift5] -> Merge/3
  [Shift4] -> Merge/4
  [Shift3] -> Merge/5
  [Shift2] -> Merge/6
  [Shift1] -> Merge/7
  [NoShift2] -> Merge/8
  [NoShift3] -> Merge/9
  ShiftFIFO_SixRight/1(Out1) -> [Shift6]
  ShiftFIFO_FiveRight/1(Out1) -> [Shift5]
  ShiftFIFO_FourRight/1(Out1) -> [Shift4]
  ShiftFIFO_ThreeRight/1(Out2) -> [Shift3]
  ShiftFIFO_TwoRight/1(Out1) -> [Shift2]
  ShiftFIFO_OneRight/1(Out1) -> [Shift1]
  NoShiftDaFIFO1/1(Out1) -> [NoShift2]
  [RxBytes] -> NoShiftDaFIFO2/1(In1)
  NoShiftDaFIFO2/1(Out1) -> [NoShift3]
  NumRxBytes/1 -> Compare To Constant19/1, Logical Operator7/3
  If/10 -> NoShiftDaFIFO2/Action
  [RxBytes] -> SwapByte1And2/1(In1)
  SwapByte1And2/1(Out1) -> [Swap1And2]
  [Swap1And2] -> Merge/10
  If/2 -> SwapByte1And2/Action
  If/3 -> ShiftFIFO_SixRight/Action
  If/4 -> ShiftFIFO_FiveRight/Action
  If/5 -> ShiftFIFO_FourRight/Action
  If/6 -> ShiftFIFO_ThreeRight/Action
  If/7 -> ShiftFIFO_TwoRight/Action
  If/8 -> ShiftFIFO_OneRight/Action
  If/9 -> NoShiftDaFIFO1/Action
  Compare To Constant6/1 -> If/9
  Logical Operator2/1 -> If/8
  Logical Operator1/1 -> If/7
  Logical Operator3/1 -> If/6
  Logical Operator4/1 -> If/5
  Logical Operator6/1 -> If/4
  Compare To Constant/1 -> If/3
  Compare To Constant17/1 -> Logical Operator9/1
  [RxByteOne] -> Compare To Constant17/1
  [RxByteTwo] -> Compare To Constant18/1
  Compare To Constant18/1 -> Logical Operator9/2
  Logical Operator9/1 -> If/2
  Compare To Constant19/1 -> Logical Operator9/3
  Compare To Constant14/1 -> Logical Operator7/1
  [RxByteOne] -> Compare To Constant14/1
  [RxByteTwo] -> Compare To Constant15/1
  Compare To Constant15/1 -> Logical Operator7/2
  Logical Operator7/1 -> Logical Operator8/2
  Logical Operator5/1 -> Logical Operator8/1
  Logical Operator8/1 -> If/1

== system HIL_Testing_SW/TX/Chiller/ChillerCmndTxDecision/CreateChillerSPCmnd/DeMuxChillerInputNumber ==
  ChillerSP_Number : Inport
  ASCIILUTable : Lookup  InputValues=[0,1,2,3,4,5,6,7,8,9]  Table=uint8([48,49,50,51,52,53,54,55,56,57]);  LookUpMeth=Use Input Nearest  OutDataTypeMode=uint8  OutDataType=fixdt(1, 16)  OutScaling=2^0  OutDataTypeStr=uint8  RndMeth=Nearest
  ASCIILUTable1 : Lookup  InputValues=[0,1,2,3,4,5,6,7,8,9]  Table=uint8([48,49,50,51,52,53,54,55,56,57]);  LookUpMeth=Use Input Nearest  OutDataTypeMode=uint8  OutDataType=fixdt(1, 16)  OutScaling=2^0  OutDataTypeStr=uint8  RndMeth=Nearest
  ASCIILUTable2 : Lookup  InputValues=[0,1,2,3,4,5,6,7,8,9]  Table=uint8([48,49,50,51,52,53,54,55,56,57]);  LookUpMeth=Use Input Nearest  OutDataTypeMode=uint8  OutDataType=fixdt(1, 16)  OutScaling=2^0  OutDataTypeStr=uint8  RndMeth=Nearest
  Abs1 : Abs  OutDataType=fixdt(1, 16)  OutScaling=2^0
  Add : Sum  Inputs=+-  OutDataType=fixdt(1, 16)  OutScaling=2^-10
  Add1 : Sum  Inputs=-+  OutDataType=fixdt(1, 16)  OutScaling=2^-10
  AsciiPoint : Constant  Value=46  OutDataTypeMode=uint8  OutDataType=sfix(16)  OutScaling=2^0  OutDataTypeStr=uint8
  AsciiS1 : Constant  Value=83  OutDataTypeMode=uint8  OutDataType=sfix(16)  OutScaling=2^0  OutDataTypeStr=uint8
  CarriageReturnAscii : Constant  Value=13  OutDataTypeMode=uint8  OutDataType=sfix(16)  OutScaling=2^0  OutDataTypeStr=uint8
  Divide : Product  Inputs=*/  OutDataType=fixdt(1, 16)  OutScaling=2^-10
  FractionPart : Lookup  InputValues=[0,.1,.2,.3,.4,.5,.6,.7,.8,.9]  Table=uint8([0,1,2,3,4,5,6,7,8,9]);  LookUpMeth=Use Input Nearest  OutDataTypeMode=uint8  OutDataType=fixdt(1, 16)  OutScaling=2^0  OutDataTypeStr=uint8  RndMeth=Nearest
  Gain{,1..6} (7 alike) : Gain  ParameterDataTypeMode=uint8  ParameterDataType=fixdt(1, 16)  ParameterScaling=2^0  ParamDataTypeStr=uint8  OutDataTypeMode=uint8  OutDataType=fixdt(1, 16)  OutScaling=2^0  OutDataTypeStr=uint8
  OnesTable : Lookup  InputValues=[0,.1,.2,.3,.4,.5,.6,.7,.8,.9]  Table=uint8([0,1,2,3,4,5,6,7,8,9]);  LookUpMeth=Use Input Nearest  OutDataTypeMode=uint8  OutDataType=fixdt(1, 16)  OutScaling=2^0  OutDataTypeStr=uint8  RndMeth=Nearest
  Output1 : Constant  Value=43  OutDataType=sfix(16)  OutScaling=2^0
  Output7 : Constant  Value=10  OutDataType=sfix(16)  OutScaling=2^0
  Output8 : Constant  Value=45  OutDataType=sfix(16)  OutScaling=2^0
  Rounding Function : Rounding  Operator=fix
  Rounding Function1 : Rounding  Operator=fix
  Sign : Signum
  Switch : Switch  Criteria=u2 > Threshold  Threshold=-1  OutDataTypeMode=uint8  OutDataType=fixdt(1, 16)  OutScaling=2^0  OutDataTypeStr=uint8
  Ascii_S : Outport  DataType=uint8  OutDataTypeStr=uint8
  PosOrNegAscii : Outport  Port=2  DataType=uint8  OutDataTypeStr=uint8
  TensDigitAscii : Outport  Port=3
  OnesDigitAscii : Outport  Port=4
  Ascii_Pt : Outport  Port=5  DataType=uint8  OutDataTypeStr=uint8
  TenthsDigitAscii : Outport  Port=6
  Ascii_CarriageReturn : Outport  Port=7  DataType=uint8  OutDataTypeStr=uint8
  wires:
  Rounding Function/1 -> Add/2, Divide/1  "ChillNumber"
  ChillerSP_Number/1 -> Abs1/1, Sign/1
  Add/1 -> FractionPart/1  "ChillFraction"
  Output7/1 -> Divide/2
  Divide/1 -> Rounding Function1/1, Add1/2
  Rounding Function1/1 -> Add1/1, ASCIILUTable1/1  "TensDigit"
  Add1/1 -> OnesTable/1
  ASCIILUTable/1 -> Gain6/1
  ASCIILUTable1/1 -> Gain5/1
  ASCIILUTable2/1 -> Gain4/1
  OnesTable/1 -> ASCIILUTable2/1  "OnesDigit"
  FractionPart/1 -> ASCIILUTable/1  "TenthsDigit"
  Output1/1 -> Switch/1
  Sign/1 -> Switch/2  "Sign"
  Output8/1 -> Switch/3
  Switch/1 -> Gain3/1
  Abs1/1 -> Add/1, Rounding Function/1
  AsciiPoint/1 -> Gain1/1
  CarriageReturnAscii/1 -> Gain2/1
  AsciiS1/1 -> Gain/1
  Gain/1 -> Ascii_S/1  "Ascii_S"
  Gain1/1 -> Ascii_Pt/1  "Ascii_Pt"
  Gain2/1 -> Ascii_CarriageReturn/1  "Ascii_CarriageReturn"
  Gain3/1 -> PosOrNegAscii/1  "PosOrNegAscii"
  Gain4/1 -> OnesDigitAscii/1  "OnesDigitAscii"
  Gain5/1 -> TensDigitAscii/1  "TensDigitAscii"
  Gain6/1 -> TenthsDigitAscii/1  "TenthsDigitAscii"

== system HIL_Testing_SW/TX/Chiller/ChillerCmndTxDecision/CreateChillerSPCmnd2/DeMuxChillerInputNumber ==
  ChillerSP_Number : Inport
  ASCIILUTable : Lookup  InputValues=[0,1,2,3,4,5,6,7,8,9]  Table=uint8([48,49,50,51,52,53,54,55,56,57]);  LookUpMeth=Use Input Nearest  OutDataTypeMode=uint8  OutDataType=fixdt(1, 16)  OutScaling=2^0  OutDataTypeStr=uint8  RndMeth=Nearest
  ASCIILUTable1 : Lookup  InputValues=[0,1,2,3,4,5,6,7,8,9]  Table=uint8([48,49,50,51,52,53,54,55,56,57]);  LookUpMeth=Use Input Nearest  OutDataTypeMode=uint8  OutDataType=fixdt(1, 16)  OutScaling=2^0  OutDataTypeStr=uint8  RndMeth=Nearest
  ASCIILUTable2 : Lookup  InputValues=[0,1,2,3,4,5,6,7,8,9]  Table=uint8([48,49,50,51,52,53,54,55,56,57]);  LookUpMeth=Use Input Nearest  OutDataTypeMode=uint8  OutDataType=fixdt(1, 16)  OutScaling=2^0  OutDataTypeStr=uint8  RndMeth=Nearest
  Abs1 : Abs  OutDataType=fixdt(1, 16)  OutScaling=2^0
  Add : Sum  Inputs=+-  OutDataType=fixdt(1, 16)  OutScaling=2^-10
  Add1 : Sum  Inputs=-+  OutDataType=fixdt(1, 16)  OutScaling=2^-10
  AsciiPoint : Constant  Value=46  OutDataTypeMode=uint8  OutDataType=sfix(16)  OutScaling=2^0  OutDataTypeStr=uint8
  AsciiS1 : Constant  Value=83  OutDataTypeMode=uint8  OutDataType=sfix(16)  OutScaling=2^0  OutDataTypeStr=uint8
  CarriageReturnAscii : Constant  Value=13  OutDataTypeMode=uint8  OutDataType=sfix(16)  OutScaling=2^0  OutDataTypeStr=uint8
  Divide : Product  Inputs=*/  OutDataType=fixdt(1, 16)  OutScaling=2^-10
  FractionPart : Lookup  InputValues=[0,.1,.2,.3,.4,.5,.6,.7,.8,.9]  Table=uint8([0,1,2,3,4,5,6,7,8,9]);  LookUpMeth=Use Input Nearest  OutDataTypeMode=uint8  OutDataType=fixdt(1, 16)  OutScaling=2^0  OutDataTypeStr=uint8  RndMeth=Nearest
  Gain{,1..6} (7 alike) : Gain  ParameterDataTypeMode=uint8  ParameterDataType=fixdt(1, 16)  ParameterScaling=2^0  ParamDataTypeStr=uint8  OutDataTypeMode=uint8  OutDataType=fixdt(1, 16)  OutScaling=2^0  OutDataTypeStr=uint8
  OnesTable : Lookup  InputValues=[0,.1,.2,.3,.4,.5,.6,.7,.8,.9]  Table=uint8([0,1,2,3,4,5,6,7,8,9]);  LookUpMeth=Use Input Nearest  OutDataTypeMode=uint8  OutDataType=fixdt(1, 16)  OutScaling=2^0  OutDataTypeStr=uint8  RndMeth=Nearest
  Output1 : Constant  Value=43  OutDataType=sfix(16)  OutScaling=2^0
  Output7 : Constant  Value=10  OutDataType=sfix(16)  OutScaling=2^0
  Output8 : Constant  Value=45  OutDataType=sfix(16)  OutScaling=2^0
  Rounding Function : Rounding  Operator=fix
  Rounding Function1 : Rounding  Operator=fix
  Sign : Signum
  Switch : Switch  Criteria=u2 > Threshold  Threshold=-1  OutDataTypeMode=uint8  OutDataType=fixdt(1, 16)  OutScaling=2^0  OutDataTypeStr=uint8
  Ascii_S : Outport  DataType=uint8  OutDataTypeStr=uint8
  PosOrNegAscii : Outport  Port=2  DataType=uint8  OutDataTypeStr=uint8
  TensDigitAscii : Outport  Port=3
  OnesDigitAscii : Outport  Port=4
  Ascii_Pt : Outport  Port=5  DataType=uint8  OutDataTypeStr=uint8
  TenthsDigitAscii : Outport  Port=6
  Ascii_CarriageReturn : Outport  Port=7  DataType=uint8  OutDataTypeStr=uint8
  wires:
  Gain2/1 -> Ascii_CarriageReturn/1  "Ascii_CarriageReturn"
  Gain1/1 -> Ascii_Pt/1  "Ascii_Pt"
  Gain/1 -> Ascii_S/1  "Ascii_S"
  AsciiS1/1 -> Gain/1
  CarriageReturnAscii/1 -> Gain2/1
  AsciiPoint/1 -> Gain1/1
  Abs1/1 -> Rounding Function/1, Add/1
  Switch/1 -> Gain3/1
  Output8/1 -> Switch/3
  Sign/1 -> Switch/2  "Sign"
  Output1/1 -> Switch/1
  FractionPart/1 -> ASCIILUTable/1  "TenthsDigit"
  OnesTable/1 -> ASCIILUTable2/1  "OnesDigit"
  ASCIILUTable2/1 -> Gain4/1
  ASCIILUTable1/1 -> Gain5/1
  ASCIILUTable/1 -> Gain6/1
  Add1/1 -> OnesTable/1
  Rounding Function1/1 -> ASCIILUTable1/1, Add1/1  "TensDigit"
  Divide/1 -> Add1/2, Rounding Function1/1
  Output7/1 -> Divide/2
  Add/1 -> FractionPart/1  "ChillFraction"
  ChillerSP_Number/1 -> Sign/1, Abs1/1
  Rounding Function/1 -> Divide/1, Add/2  "ChillNumber"
  Gain3/1 -> PosOrNegAscii/1  "PosOrNegAscii"
  Gain4/1 -> OnesDigitAscii/1  "OnesDigitAscii"
  Gain5/1 -> TensDigitAscii/1  "TensDigitAscii"
  Gain6/1 -> TenthsDigitAscii/1  "TenthsDigitAscii"
